simulink model "Mealyvendingmachine"  (R2020b)
settings: Solver=VariableStepAuto  StartTime=0.0  StopTime=10.0  RelTol=1e-3
settings Model: Creator=Shivashis  LastModifiedBy=Shivashis

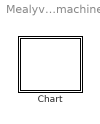
== system Mealyvendingmachine ==
  Chart : Stateflow chart  TreatAsAtomicUnit=on

== stateflow chart Mealyvendingmachine/Chart ==
